simulink model "double_track_model"  (R2021a)
settings: Solver=VariableStepAuto  StartTime=0.0  StopTime=10.0  RelTol=1e-3
settings Model: Creator=Utente  LastModifiedBy=Utente

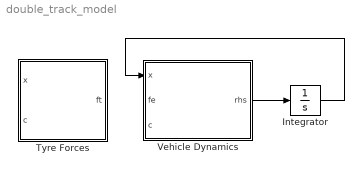
== system double_track_model ==
  Integrator : Integrator
  Tyre Forces : MATLAB Function  TreatAsAtomicUnit=on
  Vehicle Dynamics : MATLAB Function  TreatAsAtomicUnit=on
  wires:
  Vehicle Dynamics/1(rhs) -> Integrator/1
  Integrator/1 -> Vehicle Dynamics/1(x)

== matlab function double_track_model/Tyre Forces ==
  data: x input; ft output; c input; vehicle_data parameter
function ft = tyre_forces(x,c,vehicle_data)

    %extraxt slips
    alpha_rr = -(v - Omega*Lr)/u;               % assuming Wr/2*Omega << u
    alpha_rl = -(v - Omega*Lr)/u;               % assuming Wr/2*Omega << u
    alpha_fr = delta_fr - (v + Omega*Lf)/u;     % assuming Wf/2*Omega << u
    alpha_fl = delta_fl - (v + Omega*Lf)/u;     % assuming Wf/2*Omega << u
    kappa_rr = (omega_rr*rre - (u + Wr/2*Omega))/(u + Wr/2*Omega);
    kappa_rl = (omega_rr*rre - (u - Wr/2*Omega))/(u - Wr/2*Omega);
    kappa_fr = (omega_fr*rfe - (u - Wf/2*Omega))/(u - Wf/2*Omega);
    kappa_fl = (omega_fr*rfe - (u - Wf/2*Omega))/(u - Wf/2*Omega);

    %
    rear_tyre_data = vehicle_data.rear_tyre;
    front_tyre_data = vehicle_data.front_tyre;

    %call tyre force model
    Fx_rr = combined_longitudinal_force(alpha_rr,kappa_rr,gamma_rr,Fz_rr,rear_tire_data);
    Fx_rl = combined_longitudinal_force(alpha_rl,kappa_rl,gamma_rl,Fz_rr,rear_tire_data);
    Fx_fr = combined_longitudinal_force(alpha_fr,kappa_fr,gamma_fr,Fz_fr,front_tire_data);
    Fx_fl = combined_longitudinal_force(alpha_fl,kappa_fl,gamma_fl,Fz_fr,front_tire_data);

    %compute axle forces
    Fx_r = Fx_rr + Fx_rl;
    Fx_f = Fx_fr*cos(delta) - Fy_rf*sin(delta) + Fx_fl*cos(delta_fr) - Fy_rl*sin(delta_fl);

    Fy_r = Fy_rr + Fy_rl;
    Fy_f = Fy_fr*cos(delta) - Fx_rf*sin(delta) + Fy_fl*cos(delta_fr) - Fy_rl*sin(delta_fl);

    Delta_Fx_r = Fx_rr - Fx_rl;
    Delta_Fx_f = Fx_fr - Fx_fl;

end

== matlab function double_track_model/Vehicle Dynamics ==
  data: x input; rhs output; fe input; c input; vehicle_data parameter
function rhs = vehicle_dynamics(x,fe,c,vehicle_data)

    % x: vector of states
    % x = [u,v,Omega,omega_rr,omega_rl,omega_fr,omega_fl, ...
    %      Fz_rr,Fz_rl,Fz_fr,Fz_fl]
    % c: vector of inputs
    % c = [Tw_rr,Tw_rl,Tw_fr,Tw_fl,delta]
    % fe: vector of external forces
    % fe =  [FAx,FAz_r,FAz_f, ...
    %        Fx_r,Fx_f,Fy_r,Fy_f,Delta_Fx_r,Delta_Fx_f, ...
    %        Fz_rr_qss,Fz_rl_qss,Fz_fr_qss,Fz_fl_qss]
    % vehicle_data: struct with all necessary data

    %extract states
    u        = x(1);
    v        = x(2);
    Omega    = x(3);
    omega_rr = x(4);
    omega_rl = x(5);
    omega_fr = x(6);
    omega_fl = x(7);
    Fz_rr    = x(8);
    Fz_rl    = x(9);
    Fz_fr    = x(10);
    Fz_fl    = x(11);

    %extract external forces
    FAx        = fe(1);
    FAz_r      = fe(2);
    FAz_f      = fe(3);
    Fx_r       = fe(4);
    Fx_f       = fe(5);
    Fy_r       = fe(6);
    Fy_f       = fe(7);
    Delta_Fx_r = fe(8);
    Delta_Fx_f = fe(9);
    Fz_rr_qss  = x(10);
    Fz_rl_qss  = x(11);
    Fz_fr_qss  = x(12);
    Fz_fl_qss  = x(13);

    %extract from controls
    Tw_rr = c(1);
    Tw_rl = c(2);
    Tw_fr = c(3);
    Tw_fl = c(4);

    %extract parameters
    Lr    = vehicle_data.vehicle.Lr;
    Lf    = vehicle_data.vehicle.Lf;
    Wr    = vehicle_data.vehicle.Wr;
    Wf    = vehicle_data.vehicle.Wf;
    m     = vehicle_data.vehicle.mass;
    Izz   = vehicle_data.vehicle.Izz;
    rr0   = vehicle_data.wheel_rear.rr0;
    Iyw_r = vehicle_data.wheel_rear.Iyw;
    rf0   = vehicle_data.wheel_front.rr0;
    Iyw_f = vehicle_data.wheel_front.Iyw;
    tau_N = vehicle_data.vehicle.tau_N;

    % right hand side of equations of motion
    Fx_rr = Fx_r/2 + Delta_Fx_r;
    Fx_rl = Fx_r/2 - Delta_Fx_r;
    Fx_fr = Fx_f/2 + Delta_Fx_f;
    Fx_fl = Fx_f/2 - Delta_Fx_f;

    rhs(1)  = (Fx_r + Fx_f + FAx)/m + v*Omega;  %Longitudinal Dynamics
    rhs(2)  = (Fy_r + Fy_f)/m - u*Omega;        %Lateral Dynamics
    rhs(3)  = (Fy_f*Lf - Fy_r*Lr + Delta_Fx_r*Wr + Delta_Fx_f*Wf)/Izz; %missing tyre SA
    rhs(4)  = (Tw_rr - Fx_rr*rr0)/Iyw_r ;       %Wheels Equations
    rhs(5)  = (Tw_rl - Fx_rl*rr0)/Iyw_r ;       %Wheels Equations
    rhs(6)  = (Tw_fr - Fx_fr*rf0)/Iyw_f ;       %Wheels Equations
    rhs(7)  = (Tw_fl - Fx_fl*rf0)/Iyw_f ;       %Wheels Equations
    rhs(8)  = (FZ_rr_qss - Fz_rr)/tau_N;        %Vertical Loads Equations
    rhs(9)  = (FZ_rl_qss - Fz_rl)/tau_N;        %Vertical Loads Equations
    rhs(10) = (FZ_fr_qss - Fz_fr)/tau_N;        %Vertical Loads Equations
    rhs(11) = (FZ_fl_qss - Fz_fl)/tau_N;        %Vertical Loads Equations

end
